simulink model "sampleModel2016_5"  (R2023a)
settings: Solver=VariableStepAuto  StartTime=0.0  StopTime=10.0  RelTol=1e-3
libraries: hdlsllib x3, simulink x2
settings Model: Creator=user1  LastModifiedBy=user1

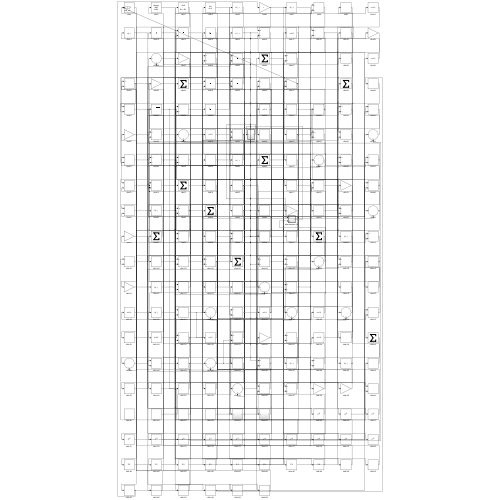
[thumbnail: Simulink's stored preview of the top-level diagram]
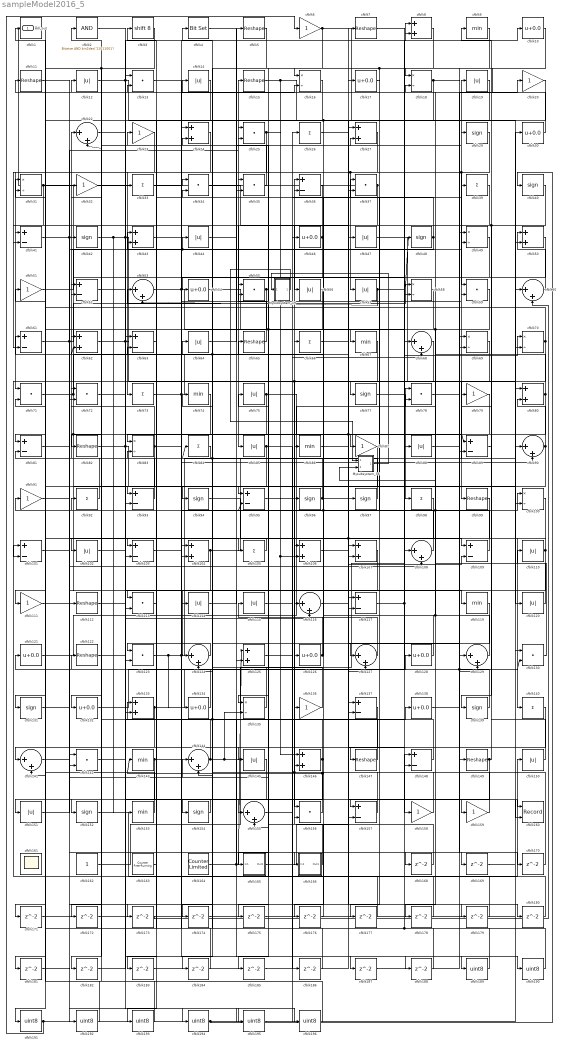
== system sampleModel2016_5 ==
  Mysubsystem_19 : Subsystem  TreatAsAtomicUnit=on  RTWFcnName=Mysubsystem_19
      settings: RTWFcnNameOpts=User specified  RTWFileNameOpts=Use function name
  Mysubsystem_36 : Subsystem  TreatAsAtomicUnit=on  RTWFcnName=Mysubsystem_36
      settings: RTWFcnNameOpts=User specified  RTWFileNameOpts=Use function name
  cfblk1 : hdlsllib/Logic and Bit Operations/Compare To Zero  relop=<=  OutDataTypeStr=uint8
  cfblk{10,17,30,46,54,121,126,128,132,134,138} (11 alike) : Bias  Bias=0.0  SaturateOnIntegerOverflow=off
  cfblk{16,18,31,49,58,69..70,83,100,135} (10 alike) : Product  Inputs=*/  OutDataTypeStr=uint8  RndMeth=Zero  SaturateOnIntegerOverflow=on
  cfblk{36,41,52,61,63,81,89,93,95,101,103,109,117,137,148,157} (16 alike) : Sum  Inputs=+-  OutDataTypeStr=uint8
  cfblk{12,14,19,44,47,56..57,64,75,85,88,102,110,114..115,120,145,150..151} (19 alike) : Abs  OutDataTypeStr=uint8  SaturateOnIntegerOverflow=off
  cfblk{8,24,27,43,50,62,80,104,106..107,125,133,146} (13 alike) : Sum  OutDataTypeStr=uint8
  cfblk{26,33,39,66,73,84,92,98,105,140} (10 alike) : Sum  Inputs=+  OutDataTypeStr=uint8
  cfblk{22,53,60,68,90,108,116,124,127,129,141,144,155} (13 alike) : Sum  Inputs=|++  OutDataTypeStr=uint8
  cfblk{5,7,11,15,65,82,99,112,122,147,149} (11 alike) : Reshape
  cfblk{6,20,23,32,51,79,87,91,111,136,158..159} (12 alike) : Gain  OutDataTypeStr=uint8
  cfblk{13,25,34..35,37,55,59,71..72,78,113,123,130,142,156} (15 alike) : DotProduct  OutDataTypeStr=uint8
  cfblk{9,67,74,86,119,143,153} (7 alike) : MinMax  OutDataTypeStr=uint8
  cfblk{29,40,42,48,77,94,96..97,131,139,152,154} (12 alike) : Signum
  cfblk160 : Record  FileSettingsInternal="{\"entries\":[{\"content\":{\"excelSettings\":{\"content\":{},\"type\":\"Streamout.ExcelSettings\"}},\"type\":\"Streamout.FileSettingStorage\",\"uuid\":\"\"}],\"packageUris\":[\"http:\\/\\/schema.mathworks.com\\/mf0\\/streamout_blocks\\/R2020a\"],\"version\":\"1.0\"}"  Layout=[1 1]  SignalsInternal="{\"entries\":[{\"content\":{\"signals\":[{\"content\":{\"blockPath\":[],\"dimensions\":[1],\"domain\":\"\",\"lineColor\":\"#a2142f\",\"plots\":[1],\"port\":1,\"signalID\":58450,\"signalName\":\"cfblk117\"},\"type\":\"RecordBlkView.Signal\",\"uuid\":\"\"},{\"content\":{\"blockPath\":[],\"dimensions\":[1],\"domain\":\"\",\"lineColor\":\"#139fff\",\"plots\":[1],\"port\":2,\"signalID\":58453,\"signalName\":\"cfblk42\"},\"type\":\"RecordBlkView.Signal\",\"uuid\":\"\"}]},\"type\":\"RecordBlkView.InputSignals\",\"uuid\":\"\"}],\"packageUris\":[\"http:\\/\\/schema.mathworks.com\\/mf0\\/streamout_blocks\\/R2020a\"],\"version\":\"1.0\"}"  VisualizationBindings="{\"xyplotplugin\":{\"info\":[{\"series\":[{\"bindingParametersList\":[{\"parameter\":\"X-Axis\",\"signalID\":58450,\"signalName\":\"cfblk117\"},{\"parameter\":\"Y-Axis\",\"signalID\":58453,\"signalName\":\"cfblk42\"}],\"seriesID\":41176}],\"subplotID\":1}]}}"  CompatibilityTag=XY  st=-1
  cfblk161 : Scope
      settings: Floating=on
  cfblk162 : Constant  OutDataTypeStr=uint8  SampleTime=-1
  cfblk163 : hdlsllib/Sources/Counter Free-Running  NumBits=16  tsamp=-1
  cfblk164 : hdlsllib/Sources/Counter Limited  uplimit=7  tsamp=-1
  cfblk165 : Subsystem
      settings: LibrarySourceBlock=|
      | hdlsllib/Ports &
      | Subsystems/Subsystem
  cfblk166 : Subsystem
      settings: LibrarySourceBlock=|
      | hdlsllib/Ports &
      | Subsystems/Subsystem
  cfblk{168..188} (21 alike) : Delay  SampleTime=1
  cfblk{189..196} (8 alike) : DataTypeConversion  OutDataTypeStr=uint8  SaturateOnIntegerOverflow=off  RndMeth=Floor
  cfblk2 : simulink/Logic and Bit Operations/Bitwise Operator  logicop=AND  UseBitMask=on  BitMask=bin2dec('11011001')  BitMaskRealWorld=Stored Integer
      settings: LibrarySourceBlock=|
      | hdlsllib/Logic and Bit
      | Operations/Bitwise
      | Operator
  cfblk3 : ArithShift  BitShiftNumber=8
  cfblk4 : simulink/Logic and Bit Operations/Bit Set  iBit=0
      settings: LibrarySourceBlock=|
      | hdlsllib/Logic and Bit
      | Operations/Bit Set
  Hdl_out : Outport  OutDataTypeStr=uint8
  wires:
  cfblk23/1 -> cfblk73/1
  cfblk51/1 -> cfblk44/1, cfblk37/2
  cfblk42/1 -> cfblk99/1, cfblk8/2, cfblk160/2, cfblk153/1
  cfblk27/1 -> cfblk57/1, cfblk61/2
  cfblk3/1 -> cfblk22/2, cfblk181/1
  cfblk94/1 -> cfblk109/1
  cfblk86/1 -> cfblk27/1
  cfblk31/1 -> cfblk93/1, cfblk41/2
  cfblk150/1 -> cfblk12/1
  cfblk72/1 -> cfblk33/1
  cfblk71/1 -> cfblk119/1, cfblk93/2, cfblk17/1
  cfblk78/1 -> cfblk129/1
  cfblk135/1 -> cfblk84/1, cfblk52/2
  cfblk166/1(Out1) -> cfblk36/1
  cfblk123/1 -> cfblk19/1, cfblk16/2, cfblk134/1
  cfblk136/1 -> cfblk64/1
  cfblk98/1 -> cfblk137/2, cfblk171/1
  cfblk65/1 -> cfblk15/1
  cfblk143/1 -> cfblk151/1, cfblk55/2
  cfblk105/1 -> cfblk102/1
  cfblk151/1 -> cfblk112/1
  cfblk24/1 -> cfblk71/1
  cfblk164/1 -> cfblk125/1, cfblk138/1
  cfblk121/1 -> cfblk78/1
  cfblk132/1 -> cfblk128/1
  cfblk47/1 -> cfblk149/1
  cfblk64/1 -> cfblk5/1
  cfblk152/1 -> cfblk150/1
  cfblk48/1 -> cfblk23/1, cfblk43/2
  cfblk99/1 -> cfblk107/2
  cfblk156/1 -> cfblk143/1, cfblk63/2
  cfblk58/1 -> cfblk142/2
  cfblk37/1 -> cfblk56/1, Hdl_out/1
  cfblk70/1 -> cfblk156/1, cfblk101/2, cfblk31/2
  cfblk19/1 -> cfblk86/1, cfblk135/1
  cfblk92/1 -> cfblk22/1
  cfblk165/1(Out1) -> cfblk47/1
  cfblk127/1 -> cfblk115/1
  cfblk142/1 -> cfblk136/1
  cfblk124/1 -> cfblk123/1
  cfblk80/1 -> cfblk104/2, cfblk52/1
  cfblk59/1 -> cfblk177/1, cfblk178/1
  cfblk85/1 -> cfblk141/1, cfblk159/1
  cfblk16/1 -> cfblk103/1
  cfblk53/1 -> cfblk108/1, cfblk59/2
  cfblk39/1 -> cfblk147/1
  cfblk17/1 -> cfblk157/1
  cfblk36/1 -> cfblk85/1
  cfblk97/1 -> cfblk35/1
  cfblk33/1 -> cfblk34/1
  cfblk34/1 -> cfblk97/1
  cfblk126/1 -> cfblk65/1, cfblk36/2
  cfblk2/1 -> cfblk194/1
  cfblk54/1 -> cfblk137/1
  cfblk100/1 -> cfblk140/1
  cfblk75/1 -> cfblk87/1, cfblk113/1
  cfblk73/1 -> cfblk26/1, cfblk8/1
  cfblk113/1 -> cfblk43/1
  cfblk159/1 -> cfblk14/1, cfblk146/2
  cfblk114/1 -> cfblk116/1
  cfblk4/1 -> cfblk190/1
  cfblk144/1 -> cfblk70/1, cfblk135/2, cfblk3/1
  cfblk60/1 -> cfblk50/1
  cfblk163/1 -> cfblk133/1
  cfblk7/1 -> cfblk158/1
  cfblk5/1 -> cfblk35/2
  cfblk30/1 -> cfblk18/1
  cfblk57/1 -> cfblk48/1, cfblk53/2
  cfblk139/1 -> cfblk122/1
  cfblk107/1 -> cfblk124/1
  cfblk133/1 -> cfblk68/1, cfblk141/2
  cfblk158/1 -> cfblk92/1
  cfblk20/1 -> cfblk103/2
  cfblk61/1 -> cfblk58/1, cfblk25/1
  cfblk154/1 -> cfblk152/1
  cfblk18/1 -> cfblk131/1, cfblk170/1
  cfblk95/1 -> cfblk30/1
  cfblk9/1 -> cfblk67/1, cfblk155/1
  cfblk155/1 -> cfblk68/2
  cfblk148/1 -> cfblk75/1
  cfblk89/1 -> cfblk9/1
  cfblk104/1 -> cfblk60/1, cfblk114/1
  cfblk102/1 -> cfblk116/2
  cfblk77/1 -> cfblk98/1
  cfblk120/1 -> cfblk18/2
  cfblk32/1 -> cfblk58/2
  cfblk44/1 -> cfblk27/2
  cfblk93/1 -> cfblk62/1
  cfblk41/1 -> cfblk55/1, cfblk113/2
  cfblk46/1 -> cfblk165/1(In1), cfblk41/1
  cfblk106/1 -> cfblk148/2
  cfblk35/1 -> cfblk11/1
  cfblk101/1 -> cfblk105/1
  cfblk110/1 -> cfblk106/1, cfblk133/2
  cfblk74/1 -> cfblk83/1
  cfblk62/1 -> cfblk120/1, cfblk180/1
  cfblk8/1 -> cfblk54/1
  cfblk87/1 -> cfblk95/1
  cfblk15/1 -> cfblk106/2, cfblk146/1, cfblk117/1
  cfblk66/1 -> cfblk29/1
  cfblk117/1 -> cfblk10/1, cfblk160/1
  cfblk79/1 -> cfblk127/1
  cfblk40/1 -> cfblk139/1, cfblk155/2
  cfblk29/1 -> cfblk59/1, cfblk72/2
  cfblk50/1 -> cfblk144/2
  cfblk69/1 -> cfblk94/1
  cfblk90/1 -> cfblk80/2, cfblk111/1
  cfblk55/1 -> cfblk81/1, cfblk145/1
  cfblk1/1 -> cfblk191/1
  cfblk67/1 -> cfblk126/1
  cfblk56/1 -> cfblk125/2, cfblk185/1
  cfblk162/1 -> cfblk109/2
  cfblk25/1 -> cfblk82/1, cfblk96/1
  cfblk153/1 -> cfblk51/1
  cfblk147/1 -> cfblk74/1, cfblk72/1
  cfblk115/1 -> cfblk39/1
  cfblk146/1 -> cfblk24/2, cfblk183/1
  cfblk26/1 -> cfblk89/1, cfblk129/2
  cfblk22/1 -> cfblk166/1(In1)
  cfblk12/1 -> cfblk90/1, cfblk188/1
  cfblk122/1 -> cfblk66/1
  cfblk140/1 -> cfblk154/1
  cfblk88/1 -> cfblk49/1
  cfblk6/1 -> cfblk89/2, cfblk16/1
  cfblk84/1 -> cfblk81/2
  cfblk129/1 -> Mysubsystem_36/2(In2), cfblk61/1
  cfblk103/1 -> cfblk100/1
  cfblk83/1 -> cfblk42/1, cfblk90/2, cfblk132/1
  cfblk130/1 -> cfblk110/1
  cfblk82/1 -> cfblk100/2, cfblk88/1
  cfblk111/1 -> cfblk108/2
  cfblk43/1 -> cfblk77/1
  cfblk128/1 -> cfblk34/2, cfblk95/2
  cfblk112/1 -> cfblk13/1
  cfblk141/1 -> cfblk49/2
  cfblk149/1 -> cfblk79/1, cfblk157/2
  cfblk108/1 -> cfblk37/1
  cfblk138/1 -> cfblk130/2, cfblk20/1
  cfblk134/1 -> cfblk121/1
  cfblk96/1 -> cfblk7/1, cfblk13/2
  cfblk109/1 -> cfblk78/2, cfblk31/1
  cfblk10/1 -> cfblk69/2
  cfblk157/1 -> cfblk53/1, cfblk62/2
  cfblk11/1 -> cfblk168/1
  cfblk168/1 -> cfblk142/1
  cfblk131/1 -> cfblk169/1
  cfblk169/1 -> cfblk70/2
  cfblk170/1 -> cfblk124/2
  cfblk171/1 -> cfblk104/1
  cfblk137/1 -> cfblk172/1
  cfblk172/1 -> cfblk50/2
  cfblk81/1 -> cfblk173/1
  cfblk173/1 -> cfblk60/2
  cfblk145/1 -> cfblk174/1
  cfblk174/1 -> cfblk107/1
  cfblk68/1 -> cfblk175/1
  cfblk175/1 -> cfblk80/1
  cfblk49/1 -> cfblk176/1
  cfblk176/1 -> cfblk156/2
  cfblk177/1 -> cfblk144/1
  cfblk178/1 -> cfblk63/1
  cfblk116/1 -> cfblk179/1
  cfblk179/1 -> cfblk101/1
  cfblk180/1 -> cfblk25/2
  cfblk14/1 -> cfblk182/1
  cfblk182/1 -> cfblk123/2
  cfblk183/1 -> cfblk117/2
  cfblk119/1 -> cfblk184/1
  cfblk184/1 -> cfblk71/2
  cfblk185/1 -> cfblk127/2
  cfblk125/1 -> cfblk186/1
  cfblk186/1 -> cfblk24/1
  cfblk52/1 -> cfblk187/1
  cfblk187/1 -> cfblk69/1
  cfblk188/1 -> cfblk83/2
  cfblk13/1 -> cfblk189/1
  cfblk189/1 -> cfblk4/1
  cfblk190/1 -> cfblk32/1, cfblk148/1
  cfblk191/1 -> cfblk6/1, cfblk46/1
  cfblk181/1 -> cfblk192/1
  cfblk192/1 -> cfblk1/1
  cfblk63/1 -> cfblk193/1
  cfblk193/1 -> cfblk2/1
  cfblk194/1 -> cfblk40/1, cfblk196/1
  cfblk91/1 -> cfblk195/1
  cfblk195/1 -> cfblk130/1
  cfblk196/1 -> cfblk91/1
  Mysubsystem_19/1(Out1) -> Mysubsystem_36/1(In1)
  Mysubsystem_36/1(Out1) -> Mysubsystem_19/1(In1)

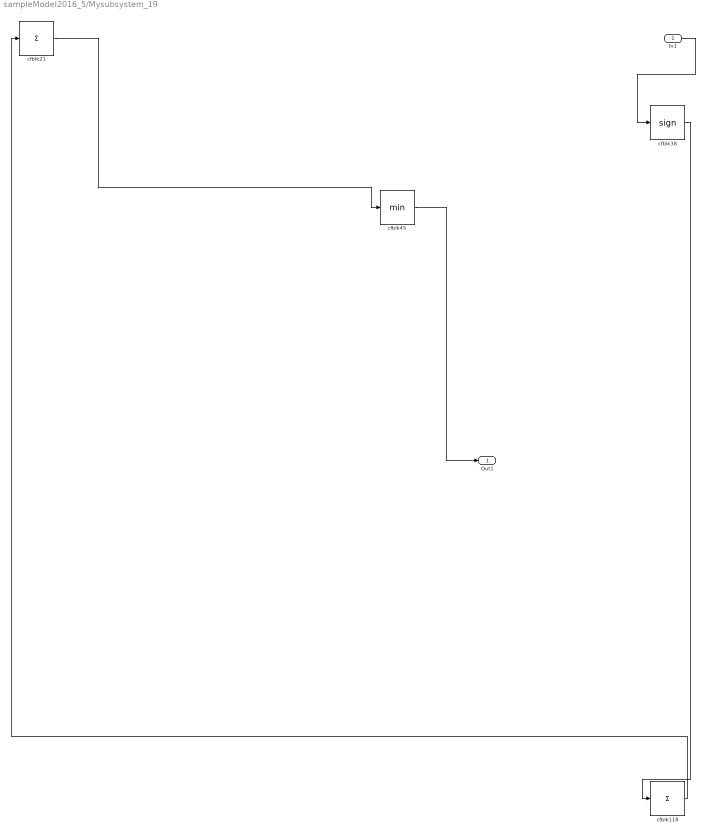
== system sampleModel2016_5/Mysubsystem_19 ==
  In1 : Inport
  cfblk118 : Sum  Inputs=+
  cfblk21 : Sum  Inputs=+
  cfblk38 : Signum
  cfblk45 : MinMax
  Out1 : Outport
  wires:
  cfblk118/1 -> cfblk21/1
  cfblk21/1 -> cfblk45/1
  cfblk45/1 -> Out1/1
  cfblk38/1 -> cfblk118/1
  In1/1 -> cfblk38/1

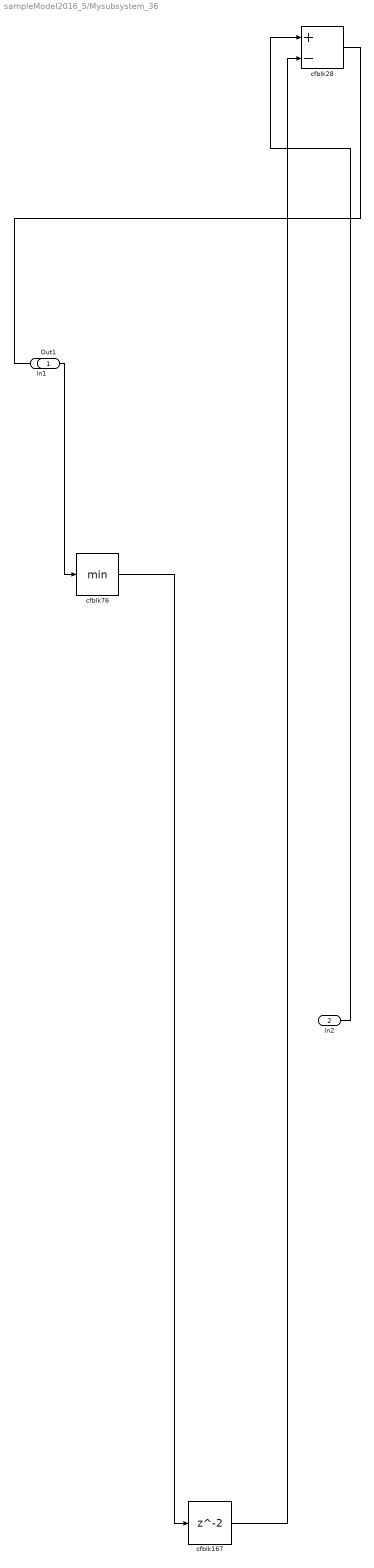
== system sampleModel2016_5/Mysubsystem_36 ==
  In1 : Inport
  In2 : Inport  Port=2
  cfblk167 : Delay  SampleTime=1
  cfblk28 : Sum  Inputs=+-
  cfblk76 : MinMax
  Out1 : Outport
  wires:
  cfblk167/1 -> cfblk28/2
  cfblk76/1 -> cfblk167/1
  In2/1 -> cfblk28/1
  In1/1 -> cfblk76/1
  cfblk28/1 -> Out1/1

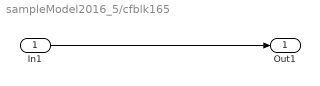
== system sampleModel2016_5/cfblk165 ==
  In1 : Inport
  Out1 : Outport
  wires:
  In1/1 -> Out1/1

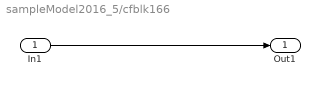
== system sampleModel2016_5/cfblk166 ==
  In1 : Inport
  Out1 : Outport
  wires:
  In1/1 -> Out1/1
